simulink model "simulacao"  (R2015a)
settings: Solver=ode45  StartTime=0.0  StopTime=10.0  RelTol=1e-3
libraries: vrlib x3
settings Model: Creator=Davi  LastModifiedBy=Davi

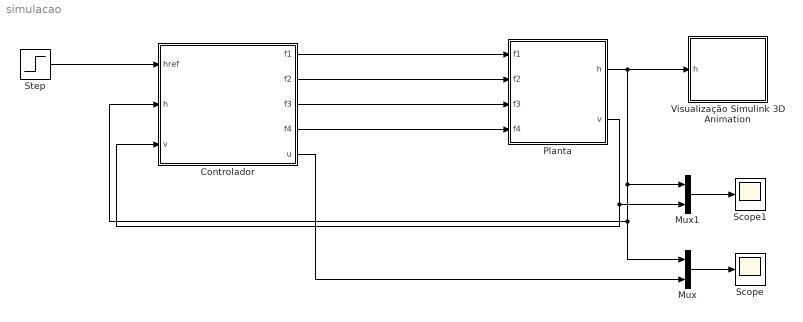
== system simulacao ==
  Controlador : Subsystem  mask{Kp=5, Kd=2, m=1, g=9.81}
  Mux : Mux  Inputs=2
  Mux1 : Mux  Inputs=2
  Planta : Subsystem  mask{m=1, g=9.81}
      mask prompts: m "massa"; g "gravidade"
  Scope : Scope
      settings: SaveName=IO  SampleInput=on  SampleTime=0.1
  Scope1 : Scope
      settings: SaveName=Estado  SampleInput=on  SampleTime=0.1
  Step : Step  SampleTime=0
  Visualização Simulink 3D Animation : Subsystem
  wires:
  Controlador/1(f1) -> Planta/1(f1)
  Controlador/2(f2) -> Planta/2(f2)
  Controlador/3(f3) -> Planta/3(f3)
  Controlador/4(f4) -> Planta/4(f4)
  Controlador/5(u) -> Mux/2
  Mux/1 -> Scope/1
  Step/1 -> Controlador/1(href)
  Planta/1(h) -> Mux1/1, Controlador/2(h), Mux/1, Visualização Simulink 3D Animation/1(h)
  Planta/2("v ") -> Mux1/2, Controlador/3(v)
  Mux1/1 -> Scope1/1

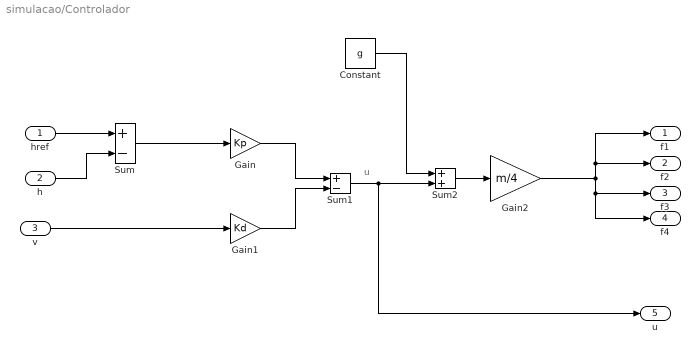
== system simulacao/Controlador ==
  note: u
  href : Inport
  h : Inport  Port=2
  v : Inport  Port=3
  Constant : Constant  Value=g
  Gain : Gain  Gain=Kp
  Gain1 : Gain  Gain=Kd
  Gain2 : Gain  Gain=m/4
  Sum : Sum  Inputs=+-
  Sum1 : Sum  Inputs=+-
  Sum2 : Sum
  f1 : Outport
  f2 : Outport  Port=2
  f3 : Outport  Port=3
  f4 : Outport  Port=4
  u : Outport  Port=5
  wires:
  h/1 -> Sum/2
  Gain/1 -> Sum1/1
  Sum/1 -> Gain/1
  href/1 -> Sum/1
  v/1 -> Gain1/1
  Gain1/1 -> Sum1/2
  Sum1/1 -> u/1, Sum2/2
  Constant/1 -> Sum2/1
  Sum2/1 -> Gain2/1
  Gain2/1 -> f3/1, f4/1, f2/1, f1/1

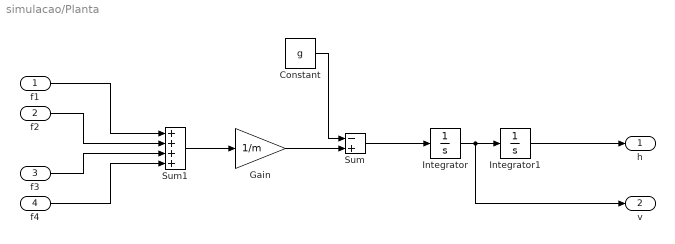
== system simulacao/Planta ==
  f1 : Inport
  f2 : Inport  Port=2
  f3 : Inport  Port=3
  f4 : Inport  Port=4
  Constant : Constant  Value=g
  Gain : Gain  Gain=1/m
  Integrator : Integrator
  Integrator1 : Integrator
  Sum : Sum  Inputs=-+
  Sum1 : Sum  Inputs=++++
  h : Outport
  "v " : Outport  Port=2
  wires:
  f3/1 -> Sum1/3
  Gain/1 -> Sum/2
  Integrator/1 -> "v "/1, Integrator1/1
  Constant/1 -> Sum/1
  Integrator1/1 -> h/1
  f2/1 -> Sum1/2
  Sum/1 -> Integrator/1
  Sum1/1 -> Gain/1
  f4/1 -> Sum1/4
  f1/1 -> Sum1/1

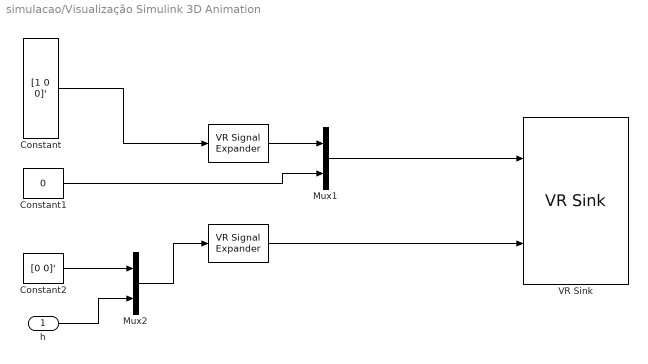
== system simulacao/Visualização Simulink 3D Animation ==
  h : Inport
  "    " : vrlib/VR Signal Expander  outwidth=3  outidx=[3 1 2]
  "      " : vrlib/VR Signal Expander  outwidth=3  outidx=[3 1 2]
  Constant : Constant  Value=[1 0 0]'
  Constant1 : Constant  Value=0
  Constant2 : Constant  Value=[0 0]'
  Mux1 : Mux  Inputs=2
  Mux2 : Mux  Inputs=2
  VR Sink : vrlib/VR Sink  InstantiateOnLoad=on  SampleTime=-1  ViewEnable=on  RemoteChange=off  RemoteView=off  FieldsWritten=Quadrotor.rotation.4.1.1.double#Quadrotor.translation.3.1.1.double  WorldFileName=Quadricopter.WRL  AutoView=on  VideoDimensions=[]  AllowVariableSize=off  FigureProperties="{'Position', 'Name', 'Viewpoint', 'CameraBound', 'CameraDirection', 'CameraPosition', 'CameraUpVector', 'ZoomFactor', 'Antialiasing', 'Headlight', 'Lighting', 'NavPanel', 'Sound', 'StatusBar', 'Stereo3D', 'Stereo3DCameraOffset', 'Stereo3DHIT', 'ToolBar', 'Textures', 'Transparency', 'Triad', 'Wireframe', 'NavZones', 'NavMode', 'NavSpeed', 'CaptureFileFormat', 'CaptureFileName', 'Record2DCompressMethod', 'Record2DCompressQuality', 'Record2D', 'Record2DFileName', 'Record2DFPS'; [5.0000000000000000e+00   9.2000000000000000e+01   5.7600000000000000e+02   3.8000000000000000e+02], '', 'Top', 'on', [0.0000000000000000e+00   0.0000000000000000e+00  -1.0000000000000000e+00], [0.0000000000000000e+00   0.0000000000000000e+00   0.0000000000000000e+00], [0.0000000000000000e+00   1.0000000000000000e+00   0.0000000000000000e+00], [1.0000000000000000e+00], 'on', 'on', 'on', 'halfbar', 'on', 'on', 'off', [1.0000000149011612e-01], [0.0000000000000000e+00], 'on', 'on', 'on', 'none', 'off', 'off', 'fly', 'normal', 'tif', '%f_anim_%n.tif', 'auto', [7.5000000000000000e+01], 'off', '%f_anim_%n.avi', 'auto'}"
  wires:
  "      "/1 -> VR Sink/2
  Mux1/1 -> VR Sink/1
  "    "/1 -> Mux1/1
  Constant1/1 -> Mux1/2
  Constant/1 -> "    "/1
  Constant2/1 -> Mux2/1
  h/1 -> Mux2/2
  Mux2/1 -> "      "/1
